simulink model "model_with_disturbance"  (R2015b)
settings: Solver=VariableStepAuto  StartTime=0.0  StopTime=5  RelTol=1e-3
values from neighbouring files (symbols this model uses):
  dg = [1 2 400]    [script.m]
  ng = 400    [script.m]
undefined symbols (not defined in the file or in its folder): denk, numk
settings Model: Creator=EriveltonDell  LastModifiedBy=EriveltonDell

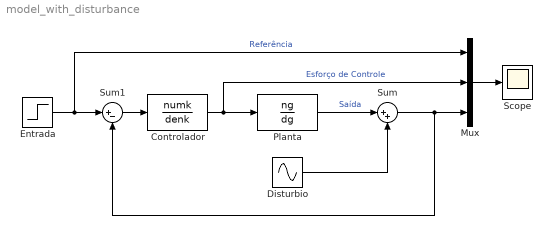
== system model_with_disturbance ==
  Controlador : TransferFcn  Numerator=numk  Denominator=denk
  Disturbio : Sin  Amplitude=0.5  SampleTime=0
  Entrada : Step  SampleTime=0
  Mux : Mux  Inputs=3
  Planta : TransferFcn  Numerator=ng  Denominator=dg
  Scope : Scope
  Sum : Sum  Inputs=|++
  Sum1 : Sum  Inputs=|+-
  wires:
  Controlador/1 -> Mux/2, Planta/1  "Esforço de Controle"
  Sum1/1 -> Controlador/1
  Entrada/1 -> Mux/1, Sum1/1  "Referência"
  Mux/1 -> Scope/1
  Sum/1 -> Sum1/2, Mux/3
  Planta/1 -> Sum/1  "Saída"
  Disturbio/1 -> Sum/2
